simulink model "Lidar_System_July11_PrintV2_Angle_Offset_Bayes_Sunny"  (Simulink 7.3)
settings: Solver=FixedStepDiscrete  StartTime=0.0  StopTime=inf  FixedStep=0.1  MaxStep=0.2  RelTol=1e-3
undefined symbols (not defined in the file): strel
libraries: dspmtrx3 x9, dspstat3 x4, simulink x3, vipstatistics x2, vipgeotforms x1, vipmorphops x1
(part 2 of 5)

== matlab function Enabled Subsystem1/Data Save Interpolation and Bayes/Bayes Filter FSM/RG Speedgate Bayes Filter ==
  data: Task input double; HMean input double; ColorProb output double; SMean input double; VMean input double; ColorNum output double
function [ColorProb, ColorNum] = BayesFilter(Task, HMean, SMean, VMean)
%Written by Anderson Lebbad on June 20, 2014
%Last Edited: by Michael Benson on 7/8/2014 for specific RG task

%Treats the histogram information as a probability distribution of the
%color of an object. Uses the Discrete Bayes Filter with the historgram
%data as measurements, starting without an input.

%initialize a variable to track previous beliefs and one to track number of
%frames iterated upon. Reset every 10 samples

persistent frames
persistent ColorProbabilities

if Task ~= 1
    ColorProb = 0;
    ColorNum = int32(0);
else
    
    if isempty(frames)
        frames = 0;
    end

    if isempty(ColorProbabilities) || frames >= 10
        ColorProbabilities = 1/2*ones(2,1);
        frames = 0;
    end

    %Histogram based probability from reference
    %Filler data from RG A2's
    Red = [0.418812802276720,0,0;0.0194722195087532,0.00139298796126768,5.07737098676741e-05;0.0138492497347506,0.00140176534989290,9.45642160859260e-06;0.0143797281837155,0.00180194953991997,1.58576916205630e-05;0.0159906356383445,0.00122250995735606,2.63324970946963e-05;0.0183249467601919,0.0568841449810760,1.03293220647704e-05;0.0218752453044534,0.00169329388232664,8.72900456177778e-07;0.0234288057788941,0.00992875149521546,9.60190501795556e-06;0.0286071400589464,0.000719431497773991,1.22206063864889e-05;0.0312588481153716,0.00160954411981461,1.97857436733630e-05;0.0305670365822222,0.00550438238362406,8.72900456177778e-06;0.0285293249011251,0.000731557411145066,3.85531034811852e-05;0.0246239069721655,0.00320793785671861,3.15698998317630e-05;0.0190959095363781,0.000679711664623136,4.23356721246223e-05;0.0171575261105718,0.00213992358772399,4.67001744055112e-05;0.0140557162320463,0.000885216251249498,3.52069850658371e-05;0.0120186805075952,0.00203428679112246,2.63324970946963e-05;0.0115340051688313,0.00271600247292672,2.63324970946963e-05;0.0103312647530754,0.00180135945137060,3.97169707560889e-05;0.00954193874440829,0.00147605615682423,3.82621366624593e-05;0.00796761104924986,0.00143910311882922,7.97249083309038e-05;0.00855603843846525,0.00169327353832533,5.95027144294519e-05;0.00739174923569342,0.00121509145857236,6.66491374325861e-05;0.00649026714238162,0.00194416565356162,6.80862355818667e-05;0.00649885840103597,0.00157160944434582,7.20231556068412e-05;0.00596040643778088,0.00194430529700334,5.70294964702815e-05;0.00540944146736658,0.00141314535097839,5.80567483079968e-05;0.00524502462779314,0.00125086331058991,5.86298139732741e-05;0.00558708173689933,0.00146083995084940,5.23740273706667e-05;0.00435272303443563,0.00144723614227691,5.44373990182717e-05;0.00549487305614555,0.00168817541534780,4.43990437722273e-05;0.00368026680360152,0.00159306007523833,6.41936554177648e-05;0.00409020974372935,0.00205652797615577,7.20586274955393e-05;0.00410089139377623,0.00167926242249156,6.27565572684842e-05;0.00326891479557737,0.00159098816892650,6.18091171803395e-05;0.00445211299670090,0.00138590680020840,5.13733794494750e-05;0.00283425405617157,0.00136777016626660,6.32107434409221e-05;0.00309300377822649,0.00140770162395038,6.94243654895015e-05;0.00307199818048493,0.00150035608420383,8.31823221224837e-05;0.00277542868469595,0.00157300356934507,6.40973915794120e-05;0.00278387992211586,0.00154389709907400,0.000110758105837365;0.00229964900594954,0.00164260827201308,7.30152979075107e-05;4.44655768338377e-05,0.00139091758695888,7.48245951759911e-05;0.00889813611845503,0.00158720488030872,8.12400052745627e-05;0.00198142826897388,0.00158792071151883,4.90456448996676e-05;0.00190651941939485,0.00180907399006750,6.19848003607968e-05;0.00225582125348853,0.00165889477609460,7.16381002566071e-05;0.00141288087150997,0.00185423950475477,6.68016758621084e-05;0.00121854137959673,0.00184987366495476,7.80571062129265e-05;0.00869650773841455,0.00198002357227974,7.90613499918661e-05;0.00283670519003113,0.00165854406467308,9.69855100676161e-05;0.0581372528555002,0.00215529068209603,8.89347029816430e-05;0.000223363632106310,0.00212468619148582,4.85581621453762e-05;0.000196405395428911,0.00200335313100036,5.16998181568990e-05;6.12350551728666e-05,0.00191817479458698,5.29736969524676e-05;0.000453580353416284,0.00186497225294572,4.70505126229886e-05;8.46548161411358e-05,0.00190663827294957,5.95825261790225e-05;0.000422587211366844,0.00199789889288887,4.79903685945255e-05;9.51697405110890e-05,0.00221563798239625,5.55643738535741e-05;6.97094055950642e-05,0.00226156124634891,4.37469211133207e-05;0.000352672020849422,0.00250472020727048,4.08346852181048e-05;0.000106693307556525,0.00241527118012696,3.37179629390762e-05;7.61772640109071e-05,0.00258882988304447,2.83021726150822e-05;6.65529572666487e-05,0.00196684177186773,4.15487469837195e-05;8.60084106627102e-05,0.00233772119111424,5.40230353450440e-05;4.93082961912820e-05,0.00227698508497096,6.21985231410858e-05;6.99871626200540e-05,0.00236118701349608,7.77381149267738e-05;4.17810794906234e-05,0.00243959790993590,6.65413012187658e-05;9.43059460511410e-05,0.00262381505622098,6.25955132216168e-05;4.39327384493303e-05,0.00241272700598437,7.11457377921782e-05;6.77317370658152e-05,0.00242356907176823,5.06884893083404e-05;8.80904909050683e-05,0.00234279285042164,4.30549459025671e-05;4.10054710162356e-05,0.00202206116654657,5.70360223908153e-05;5.25969928584074e-05,0.00253828795216140,6.09308079112216e-05;5.98094799256230e-05,0.00250010189524607,6.65882087875949e-05;5.27204786738887e-05,0.00246939421035033,7.97439281308196e-05;5.88503183894037e-05,0.00237587522755561,9.40260932097212e-05;7.13108537607895e-05,0.00239990545025178,8.51284604812913e-05;6.99192479465926e-05,0.00253939132480483,7.10672098981744e-05;6.26092432317400e-05,0.00246119719969018,5.85516484309226e-05;7.76478903519452e-05,0.00256105193836888,7.05681848178752e-05;4.72027776745463e-05,0.00287320739593677,5.61533324585485e-05;6.22308504878448e-05,0.00278061158556548,5.36609880535855e-05;7.84365984049347e-05,0.00319713203504958,3.84505093291548e-05;2.54326892786854e-05,0.00185097795461185,4.59198818278418e-05;0.000151473372383540,0.00271584846618697,3.32438054165253e-05;2.80180039138091e-05,0.00274595292638483,3.93912567519695e-05;5.53332462627916e-05,0.00260298523939083,3.34981354982484e-05;3.61831896348111e-05,0.00263263624778821,3.35821788510691e-05;5.77372432354937e-05,0.00271640119762721,3.17842872132601e-05;5.27135797825679e-05,0.00267032135785430,4.02966389351400e-05;5.05695379036930e-05,0.00268493871523649,3.49858737726195e-05;9.54953413418300e-05,0.00264011882154095,2.89231439463432e-05;6.33501539846335e-05,0.00290170646338386,3.95766693095964e-05;5.50300412672821e-05,0.00283048196980252,4.13286938897529e-05;8.29360851845888e-05,0.00246888746902639,4.71112745231836e-05;3.19810588641323e-05,0.00267918261210111,6.12189501224616e-05;5.23961728497560e-05,0.00274481937827211,6.51297788425716e-05;3.86472632951297e-05,0.00262356594581976,6.53501341892712e-05;5.22572754598462e-05,0.00271370327253989,7.01879791346731e-05;4.60110638382893e-05,0.00275933382763916,7.20086054437621e-05;6.99936331887945e-05,0.00223294619925761,6.72752141398318e-05;6.34334042725368e-05,0.00278169157892946,8.54299279338030e-05;4.38411398324308e-05,0.00279272622079914,8.12459885466860e-05;9.43428590703418e-05,0.00269523707432427,6.17352722085717e-05;4.49809708955904e-05,0.00274871566290032,7.91683701666031e-05;0.000101528135318529,0.00261970779585040,7.44322579682364e-05;4.57463863187916e-05,0.00291387702632575,8.30153401757590e-05;0.000101998442490373,0.00300732388907046,7.40743656836110e-05;8.41092087030208e-05,0.00262624994339149,8.07877210278278e-05;0.000141195946627944,0.00274473037832307,8.91614776125309e-05;0.000127079022997702,0.00270019219328425,8.80237753092585e-05;0.000104131277246489,0.00273021498477153,0.000103968333693197;0.000156109716199346,0.00251020137785535,9.53120858671849e-05;0.000119420105949319,0.00269722007726919,8.52350252231697e-05;0.000153257388529412,0.00244661861602097,6.89965399019053e-05;0.000136609073394080,0.00294979261554324,7.26876177839587e-05;0.000155567767174597,0.00261027159125617,7.14209306975316e-05;0.000113628465885678,0.00285682877063998,8.11734545471175e-05;0.000125949367977156,0.00275960592382486,7.48608642568922e-05;0.000189291966171453,0.00290114176043710,7.82491171704545e-05;0.000210477071818512,0.00278464363993004,6.90690232533521e-05;0.000247727879635590,0.00287502885651961,7.24844091798863e-05;0.000221224323355267,0.00286507033400682,8.56833035452100e-05;0.000247606435361267,0.00305545204943198,6.77579963028754e-05;0.000390223396282197,0.00266116362026216,6.35203500357226e-05;0.000463359252947279,0.00291547128955731,7.05580453769359e-05;0.000316948843843813,0.00135623585761069,7.51642949055405e-05;0.000303566796056351,0.00263290137599010,7.01890497048407e-05;0.000100012530563643,0.00270369869106788,8.81672024349243e-05;0.000144023951274503,0.00267933701167384,8.05940886207993e-05;0.000131935473019354,0.00268146392101225,0.000108123357171141;9.93491089135877e-05,0.00268449853401116,0.000112412291673449;4.11202732797045e-05,0.00259712269173432,0.000117932821400504;3.20593145643942e-05,0.00254079690907548,0.000118166954469444;2.02291422820886e-05,0.00233601609979998,0.000134378972572698;2.05342491905928e-05,0.00270755173260891,0.000141445084785627;1.50928830935123e-05,0.00217625541337369,0.000149639455686249;1.30206434737328e-05,0.00259279807425540,0.000176067021727887;9.38715409422949e-06,0.00230652974475116,0.000174625858736038;7.05055157224756e-06,0.00251745490097623,0.000163270705387633;3.89785228170570e-06,0.00241470223741854,0.000158378761154729;2.65417325723139e-06,0.00252839483583534,0.000146063703891434;5.68799305493382e-06,0.00229740754916477,0.000141062639592320;8.81768428352291e-07,0.00244158084725999,0.000139490994673173;2.57076565309001e-06,0.00219131267591570,0.000130534762983653;1.47257003797866e-06,0.00247860264745366,0.000148967327526605;2.69851311810395e-06,0.00238203133567418,0.000141371960412823;1.37142648948826e-06,0.00200835386214405,0.000151771590515841;0,0.00207035940930703,0.000136619032573913;6.49173263627104e-06,0.00222783724179691,0.000152182536243749;0,0.00211111991830051,0.000142728819044803;1.19933916360175e-06,0.00176935628873998,0.000171308722220559;1.45483409362963e-07,0.00223939320858555,0.000184828783178880;3.03381979770244e-06,0.00217074353330532,0.000183863880543413;1.45483409362963e-07,0.00205145924617477,0.000197484841709011;0,0.00184969041659710,0.000189521008029114;1.18160321925273e-06,0.00203302391019745,0.000185315118782472;0,0.00205057741964801,0.000203145053647263;7.36285018989328e-07,0.00191872611987478,0.000201114234986847;0,0.00227938125138302,0.000195226313365008;3.09949145749479e-06,0.00212336341397899,0.000213486125996751;0,0.00205412921341422,0.000207473566094751;2.99834790900439e-07,0.00185151516359060,0.000207406521624767;8.90636400526803e-07,0.00186248859732819,0.000183341482655647;1.68899722473772e-06,0.00193500038779790,0.000211978261985679;0,0.00199879299929424,0.000196068363552520;0,0.00213005077179156,0.000213310677211431;1.45483409362963e-07,0.00226448101068235,0.000254057130439161;0,0.00157666277757647,0.000266568758413429;0,0.00240265450950301,0.000285630735682664;9.53352895487022e-06,0.00212217380237139,0.000316744144969953;0,0.00217033136797276,0.000347296809278156;0,0.00195155596397510,0.000350819310353655;0,0.00197136585358172,0.000374224667783579;0,0.00197401567470083,0.000333386251171196;0,0.00225727278194117,0.000376045619823585;4.63054144612427e-07,0.00225500699055331,0.000413333437163438;4.54186172437914e-07,0.00206219785523074,0.000407191651543640;2.99834790900439e-07,0.00214402826730192,0.000456285295707928;0,0.00210716655790327,0.000463388104092460;9.08372344875829e-07,0.00224111576073664,0.000492907406114772;0,0.00170207435823317,0.000490017162461332;7.71756907687378e-07,0.00207988071440082,0.000479532398573352;0,0.00201065397987837,0.000516543874663399;2.98947993682987e-06,0.00199450170188781,0.000464866534941865;0,0.00177671736127319,0.000469246302623159;1.45483409362963e-07,0.00189175987991769,0.000527230176751719;1.54351381537476e-07,0.00187401189637039,0.000600250030866361;9.26108289224854e-07,0.00200277400075776,0.000514808246628158;0,0.00197953547678507,0.000562698936262369;0,0.00155455061017225,0.000572964589360564;4.22518244040745e-06,0.00198779350468226,0.000523625276904511;0,0.00200076476505620,0.000616447190540555;1.54351381537476e-07,0.00176354543818283,0.000642568677493060;0,0.00201458246429843,0.000632021564242528;9.26108289224854e-07,0.00198485552332751,0.000689386452587112;0,0.00188631273418289,0.000684597701362130;0,0.00194984914991706,0.00104741783900229;2.41641427155253e-06,0.00186793794617886,0.00100164960594678;0,0.00189473075595684,0.000959830770760674;3.08702763074951e-07,0.00190594993204555,0.00112452932795823;0,0.00194085676172101,0.00101608491830048;1.31821865644118e-06,0.00170847754263923,0.00108169844026045;0,0.00198170260629892,0.00105383542393514;3.08702763074951e-07,0.00210488869443961,0.00102225981496908;4.63054144612427e-07,0.00196488951978371,0.00142330496824817;1.54351381537476e-07,0.00196396824180039,0.00140267367413510;0,0.00190308572363885,0.00120878275630225;0,0.00187071228421696,0.00205322784788965;0,0.00198115641717238,0.00173893426378925;0,0.00208977844254468,0.00188806599530812;0,0.00179340738821397,0.00167046248806787;1.24298418641064e-05,0.00218935197268131,0.00275908125480616;0,0.00192774256781834,0.00157355834898318;0,0.00204901563154405,0.00350939920376686;0,0.00202326008635860,0.00632085665053410;0,0.00213558501768675,0.00669789463168136;1.08045967076233e-06,0.00207714353839267,0.00627563514000161;0,0.00225995513740419,0.00250544981401045;1.45483409362963e-07,0.00223563601660356,0.00628662925532504;0.000107410825605734,0.00228770076342562,0.00694054742809225;2.13431542500112e-06,0.00225603417304346,0.00563315640424600;2.90966818725926e-07,0.00220257190544410,0.00749520898429996;2.67190920158041e-06,0.00222918142788297,0.0101271846978441;2.99834790900439e-07,0.00234595332802456,0.00694290376571382;1.49030598232768e-06,0.00229601957392332,0.0129468824474908;8.90636400526803e-07,0.00258945498766694,0.0159801589818961;4.27093165619752e-05,0.00230717065782069,0.0150667035339748;1.31821865644118e-06,0.00237610367689422,0.0144312222281109;3.11722740184381e-06,0.00240501038018950,0.0387860160710828;6.85186032983753e-06,0.00230587982511823,0.0142080286927282;5.00851172356233e-06,0.00240837658981136,0.253900841876681;4.50998569025186e-06,0.00258880916558226,0.0183449808209977;4.99964375138782e-06,0.00265683863733496,0.0144575158948879;3.75555647575547e-05,0.00342846223898661,0.0170167582050570;1.74294856154943e-05,0.00331827817329332,0.0171418698632039;1.37299321687324e-05,0.00339160394932691,0.0174772463377933;1.16501084323452e-05,0.00383120615703546,0.0178604644454266;2.10577028773938e-05,0.00404692001829078,0.0196329380603643;2.43128295719929e-05,0.00436779279654884,0.0212313110641294;4.08217347279958e-05,0.00609041339337509,0.0228963122790907;3.85503035932928e-05,0.00632406275849346,0.0227626430174866;2.26835183505936e-05,0.00663320374789515,0.0254917960021599;3.32935187110122e-05,0.0156813466261263,0.0244074642420541;4.90044365398483e-05,0.0242377204839236,0.0238488375177945;3.74385382082969e-05,0.0254873378699169,0.0202960165575666;3.70503572106603e-05,0.287237951700180,0.0201973404850723;5.25056022033951e-05,0.00590919265813658,0.0192098345312769;9.09691580564597e-05,0.0135465726949558,0.0195085996911853;0.000121508740524264,0.00247847860111233,0.0161886324548659;0.000301689558076566,0.00212561673317700,0.0147470760761275;0.000480987078225832,0.00136429432132458,0.0153705482830582;0.00116738829366397,0.00105211487702614,0.0727297039365956;0.0112209100765555,0.00644597379873206,0.0532084254345464;0,0,0];
    Green = [5.64759498395346e-05,0,0;8.59416627992918e-06,2.45547607997977e-05,0;1.90299396198432e-05,0.000189685527178437,0;7.55058894593778e-05,0.00117801464937029,6.13869019994942e-07;0.000150397909898761,0.000844683771513040,0;9.14664839792463e-05,0.00123633220626981,3.68321411996965e-06;0.000142417612638826,0.00105892405949127,4.29708313996459e-06;0.000142417612638826,0.000675255921994436,2.51686298197926e-05;0.000230200882498103,0.000716999015354092,2.94657129597572e-05;5.58620808195397e-05,0.000726207050654016,7.61197584793728e-05;0.000174952670698558,0.000755672763613773,3.37627960997218e-05;0.000307548379017466,0.000762425322833718,4.54263074796257e-05;0.000289420246980742,0.000736028954973935,3.58923417228313e-05;0.000283281556780793,0.000649473423154648,3.83478178028111e-05;0.000301947574050020,0.000649473423154648,4.87835911427251e-05;0.000237779265513676,0.000776544310293601,3.40507346628465e-05;0.000173361010307953,0.000828109307973176,7.42401595256423e-05;0.000331261319434795,0.000915892577832453,5.21788666995701e-05;0.000165804622599285,0.000850822461712989,0.000112799932104087;0.000142515591733223,0.000728662526733996,0.000107964963731619;0.000126077099181502,0.000774088834213622,0.000156172677748094;0.000280310190775215,0.00100981453789168,0.000176104424951057;0.000179141776877351,0.00102884447751152,0.000198567632021491;0.000183416864710410,0.000995081681411801,0.000159893883761809;0.000187561980275393,0.000963160492372064,0.000188093866787831;0.000176126420257962,0.000984645908071887,0.000233808112830582;0.000169699791494888,0.000979121086891932,0.000234134043287452;0.000165152761685545,0.000940447338632251,0.000341735084668454;0.000275899131954013,0.00103158789215463,0.000340545338522210;0.000205804087993353,0.000976627618918207,0.000348085729644037;0.000196997966937790,0.000945858184130968,0.000355028248332710;0.000167972160116140,0.000945532253674098,0.000319885746618016;0.000253761855340450,0.00109054131338105,0.000496392085813434;0.000193102798042187,0.00119077592652211,0.000510571060473969;0.000251958240174211,0.000954822271481579,0.000559756565861055;0.000292821521257652,0.00100104240958315,0.000399460767854884;0.000216603783683883,0.000802262822786028,0.000345462289402235;0.000247433205671772,0.00112734746012713,0.000326954238428055;0.000271374097451575,0.00105585071524459,0.000470067702594433;0.000214132311017063,0.000976313685901467,0.000380170883698887;0.000255799420589228,0.00102051225534110,0.000468302079321939;0.000195814219511611,0.00120690048605709,0.000382262437428251;5.46343427795498e-05,0.00122639232712195,0.000474576740510031;0.000634540609339266,0.00120941594933772,0.000488929678052453;0.000230402839406961,0.00127995089943649,0.000496432077280535;0.000306788541142554,0.00139554823466427,0.000576544983749907;0.000232276439640627,0.00107708018555497,0.000476190396207542;0.000381278647337575,0.00125351054096290,0.000658461505385519;0.000403187972588665,0.00128177051118957,0.000565849265873839;0.000451873584636993,0.00120901803424007,0.000655072228548739;0.000473472976018053,0.00147160200722292,0.000658733447361803;0.000478671866741137,0.00150686448333892,0.000719778422317587;0.000394169896757469,0.00146907654607552,0.000708184896005109;0.000446984627783939,0.00155343254720427,0.000867698860829463;0.000383484176748176,0.00165554675929906,0.000687889226451530;0.000318300084947475,0.00148379340596856,0.000647765787509451;0.000330577465347374,0.00148435928522803,0.000645038369453187;0.000727000881275964,0.00169511231727509,0.000608924075087947;0.000416845058603536,0.00166131752800169,0.000503936476081971;0.000389872813617504,0.00179897215690882,0.000514638192678105;0.000464476895493762,0.00182383685157865,0.000661174926428298;0.000589940125655269,0.00182472266257493,0.000630039569717089;0.000625148613290679,0.00182507258791206,0.00100136834004002;0.000750883785428471,0.00159226826090571,0.000557341081248176;0.00109448847118388,0.00189448977650537,0.000580316179097498;0.000913545078713645,0.00207851651108906,0.000418236761658638;0.00103039814600838,0.00216843532529151,0.000525267924633457;0.00123675611582108,0.00226885989790130,0.000374706049719583;0.00168685807846551,0.00262634762146070,0.000329915606566858;0.00210315525396977,0.00263831906713728,0.000310559736490145;0.00238629284146900,0.00270115366024582,0.000276606980921695;0.00273374270678614,0.00255027185359514,0.000275705173338575;0.00279548953198954,0.00267357354495986,0.000320599594305762;0.00372449131273758,0.00295677911795316,0.000381584582060895;0.00487414401364010,0.00298961411201615,0.000429814291384276;0.00514913134014422,0.00286661635580140,0.000472975082252650;0.00569852411730614,0.00282401944461914,0.000615186738835908;0.00815310038927614,0.00330093168680785,0.000720202331868854;0.0107508621100533,0.00271035769639904,0.000653366592476897;0.0115851920907340,0.00328122189224730,0.000633918742025852;0.0129208710995752,0.00336854725980827,0.000759473952561690;0.0153363777077613,0.00311447946974450,0.000764488882536111;0.0193231670544919,0.00336194266901660,0.000708648797023477;0.0214687792495091,0.00330959383858185,0.000838291135497001;0.0255558092081009,0.00254408917278138,0.000688787034887940;0.0774038724905344,0.00347457663653222,0.000884309316689717;0.0413451982577381,0.00313356339784493,0.000861360213294010;0.0338858518435638,0.00356296577711807,0.000977741381276960;0.0301487272263692,0.00324231019475837,0.000817907484715801;0.0306436356287532,0.00325953451963861,0.00108866371400067;0.0332230312682644,0.00367098872847698,0.00111743557500623;0.0374729024817433,0.00364719180597874,0.00113174852108155;0.0397526880484565,0.00340957450590682,0.00121187742413777;0.0378740048993227,0.00349219087821670,0.00114813702429940;0.0324405302289461,0.00340957050676011,0.00135120969508978;0.0290666781010269,0.00342488923823302,0.00136713029814255;0.0296407496125367,0.00402534911930911,0.00145728906114760;0.0356849959637812,0.00483235493009328,0.00157320432853883;0.0395630245165850,0.00437495852384968,0.00216359435819898;0.0407753598430210,0.00424826955522154,0.00160306195787617;0.0380115275563884,0.00498365264800180,0.00154762978532796;0.0368282500299476,0.00354253613614970,0.00173022282581610;0.0298285795356416,0.00453824568359498,0.00184178502201342;0.0210234802620634,0.00409398047557389,0.00244841958560986;0.0164048057394090,0.00364579410420357,0.00298893225750208;0.0110889379754820,0.00403142982188177,0.00338672938032558;0.00908992650056243,0.00426539990015410,0.00347458863397235;0.00814236268035962,0.00379832955801887,0.00359348926438264;0.00720789806520562,0.00399952462942887,0.00441631969869853;0.00639686311411107,0.00335357445452579,0.00372866442232954;0.00608482769248491,0.00376550256224930,0.00491582312065239;0.00572428861998573,0.00361931575383624,0.00333207504181248;0.00615469278550974,0.00392753598950099,0.00435011382491341;0.00583404720101681,0.00396643968869650,0.00353824505172980;0.00481320501607213,0.00425503011273491,0.00490912654948639;0.00461989626197437,0.00435664443149094,0.00484768765857967;0.00432509116394853,0.00436277512339747,0.00482097135898308;0.00428296615207806,0.00417634890078774,0.00561831723088908;0.00444561344834975,0.00412345618640042,0.00479221749413771;0.00485890926424811,0.00399275807319544,0.00541906774435352;0.00455306652130248,0.00426289643431360,0.00456264647724644;0.00445239200202331,0.00371740082562064,0.00514094308725536;0.00292324427321591,0.00381317639017998,0.00458484774020737;0.00228359275438118,0.00371428549033350,0.00516145271115793;0.00206628312130297,0.00351831730367355,0.00523129580887585;0.000976665610811952,0.00422639422271749,0.00480587058100587;0.000291587784497597,0.00461505529488184,0.00559332656309789;7.91891035793475e-05,0.00283711465052125,0.00483196501328904;8.53277937792969e-05,0.00437326288564462,0.00601825789634917;1.22773803998988e-06,0.00408650607037278,0.00495514673025246;5.52482117995448e-06,0.00400633717584946,0.00554387111530787;2.51686298197926e-05,0.00408818171284429,0.00567739662523687;2.27131537398128e-05,0.00398538764580879,0.00608597144844399;6.75255921994436e-06,0.00380842940303513,0.00558363463104604;9.20803529992413e-06,0.00384641129891397,0.00604918729700481;9.20803529992413e-06,0.00372969820175409,0.00621786330694192;9.20803529992413e-06,0.00400794083368020,0.00606026093424498;6.75255921994436e-06,0.00380664578360244,0.00669104834439685;4.91095215995953e-06,0.00358835036086020,0.00605819537496923;3.06934509997471e-06,0.00360229738501155,0.00596688685728503;6.13869019994942e-07,0.00382027287601699,0.00535548930995691;1.22773803998988e-06,0.00353426790032664,0.00576435607087387;0,0.00335357845367250,0.00644283730468997;0,0.00337721740987569,0.00604661584567024;6.13869019994942e-07,0.00348590621916183,0.00699461157371774;0,0.00342531714693099,0.00635565390683721;0,0.00372344753544626,0.00619957920818351;0,0.00347543045435482,0.00658468703849597;0,0.00366662365984295,0.00592171649519485;0,0.00356604711965817,0.00645419688091991;1.22773803998988e-06,0.00406898380906263,0.00567350145634126;0,0.00448059198504933,0.00693635800316558;0,0.00382477591521252,0.00621570576729184;0,0.00485564995967940,0.00668098449170098;0,0.00517649750108119,0.00584956788939857;0,0.00467551439484460,0.00502189248884344;0,0.00470294254255558,0.00603507630783835;6.13869019994942e-07,0.00552914425754806,0.00536562514729357;0,0.00472664748467949,0.00753366455706079;0,0.00517075072725883,0.00610449549600501;0,0.00517506380698563,0.00765498067208396;0,0.00434342525204082,0.00595371766716879;0,0.00474935463969924,0.00645238526746025;0,0.00471952700396222,0.00584119767533441;0,0.00432027819088297,0.00574709575367323;0,0.00484209285233228,0.00581612102588895;0,0.00462894233183254,0.00493404123349009;0,0.00456246051692442,0.00575447817850001;0,0.00473505769021076,0.00554162559443017;0,0.00386035432391861,0.00732101193032645;0,0.00599809619821038,0.00634392640910994;0,0.00479977788099309,0.00704802417717736;0,0.00466920774048283,0.00625805473137808;0,0.00440997905158972,0.00624668115813465;0,0.00465340111311130,0.00624744699472963;0,0.00439547214689896,0.00589866341398469;0,0.00439056919303242,0.00600098558170840;0,0.00443649139470410,0.00569505485753516;0,0.00431867253347888,0.00691925765183334;0,0.00421240320795233,0.00662945348676844;0,0.00467333485988762,0.00705019171469422;0,0.00447672281060735,0.00597042010340338;0,0.00395828742812804,0.00623599143897865;0,0.00482459858504911,0.00539866009869206;0,0.00454055319124669,0.00583414118096450;0,0.00432886035972277,0.00486946501198932;0,0.00410780752532394,0.00582520308806751;0,0.00422122332602137,0.00548064260624839;0,0.00439713979107706,0.00544155894545093;0,0.00428031071866258,0.00533965668813177;0,0.00470300053018288,0.00525706830984886;0,0.00393274687766421,0.00520099427425369;0,0.00555682835064848,0.00487591563563266;0,0.00457001690463309,0.00531875714742497;0,0.00420474884114926,0.00495514273110575;0,0.00465595856743238,0.00519652322823184;0,0.00463093190732080,0.00500288454453050;0,0.00492873236623248,0.00567429128781650;0,0.00419772034080632,0.00489002262565241;0,0.00421868386786048,0.00526393884389676;0,0.00511469268825049,0.00488106053787516;0,0.00526538453543245,0.00467656817000270;0,0.00490855467150685,0.00456539389103626;0,0.00345000987829229,0.00406302308089128;0,0.00462860640350890,0.00453736787089212;0,0.00456198261889257,0.00404162364684572;0,0.00493546293014552,0.00444073448936347;0,0.00467908963200340,0.00422475257299301;0,0.00431227789788948,0.00444271006783825;0,0.00409613001693055,0.00467503049809268;0,0.00461236786829268,0.00474394579377387;0,0.00445775885690822,0.00499614998147075;0,0.00446023832786846,0.00474439969692547;0,0.00442528378604914,0.00438825968580736;0,0.00448351736086775,0.00423129117786396;0,0.00422702608789768,0.00380091500636692;0,0.00387561106861751,0.00360495081885368;0,0.00415454955207117,0.00351548590780282;0,0.00432765461698968,0.00405649247431374;0,0.00442837912560273,0.00426218858534592;0,0.00455286256482027,0.00456368025667100;0,0.00571846186322917,0.00474052852291012;0,0.00489332192168821,0.00501781735834589;0,0.00554325124756781,0.00511884980125561;0,0.00539161360218893,0.00499287468031521;0,0.00647129923182551,0.00466519459675928;0,0.00636939897407970,0.00441318636725119;0,0.00595304181137479,0.00406295109625050;0,0.00726374015029161,0.00375835808665177;0,0.00718969594895476,0.00381996294214696;0,0.00701155595832828,0.00382337621386400;0,0.00928017990657369,0.00394267875851865;0,0.0100841063743911,0.00444330794027140;0,0.0117657975553072,0.00452831980146060;0,0.0148302077082417,0.00453800173564567;0,0.0193894089205974,0.00453077327796723;0,0.0178914325408216,0.00495280522985372;0,0.0176311900682375,0.00464262341272767;0,0.0178718387215157,0.00506823460091967;0,0.0170407240547899,0.00615487874583176;0,0.0155849946608592,0.00678355260694736;0,0.0125271870991430,0.00828430839368666;0,0.0100083805318627,0.00895988224784454;0,0.00969168610431929,0.0101424999150781;0,0.00543921344590547,0.0115618850637077;0,0.00547018083845486,0.0133732605741378;0,0.00277857314140596,0.0144005813767528;0,0.00380991708561128,0.0166686794372058;0,0.00173858704116020,0.0182121861022757;0,0.00213851570918016,0.0186627399684984;0,0.00181987169761562,0.0195606703788826;0,0.00113063075957609,0.0184694192169605;0,0.00161016844157996,0.0154263585087377;0,0.000453611213882516,0.0122882820738305;0,0.0290299159448947,0.0333400223061206;0,0,0];
    

    RedH = Red(:,1);
    RedS = Red(:,2);
    RedV = Red(:,3);
    GreenH = Green(:,1);
    GreenS = Green(:,2);
    GreenV = Green(:,3);

    %Combine probs into channel matrices
    ProbH = [RedH, GreenH];
    ProbS = [RedS, GreenS];
    ProbV = [RedV, GreenV];

    %No input, 2 measurements, 2 states
    for i=1:2
        ColorProbabilities(i) = (ProbH(HMean+1,i)*ProbS(SMean+1,i)*ProbV(VMean+1,i))*ColorProbabilities(i);
    end

    %Sum for normalization
    TotalProb = sum(ColorProbabilities);

    %Update frame count
    frames = frames + 1;

    %Check to make sure ColorProbabilities has values, if so normalize
    if (TotalProb == 0)
        ColorProbabilities = 1/2*ones(2,1);
        frames = 0;
    else
        %Normalize
        ColorProbabilities = ColorProbabilities/TotalProb;
    end



    %Output - First element is red prob, then green prob
    [OrderedProbs, Order] = sort(ColorProbabilities,'descend');
    ColorProb = OrderedProbs(1);
    %ColorProb = 0.6;
    ColorNum = int32(Order(1));
end

== matlab function Enabled Subsystem1/Data Save Interpolation and Bayes/Template Matching Subsystem/Detection/Detection ==
  data: cruciform input double; bbox_out output double; circle input double; triangle input double; whitePixCount input double; threshold input double; V_mask input double; bbox_in input double; label input double; rtnRatioDiff output double
function [bbox_out,rtnRatioDiff]= detection(cruciform,circle,triangle,...
    whitePixCount,threshold,V_mask,bbox_in,label)

% Written by Edward Zhu on 5/14/14
% Last Edited by Anderson Lebbad on 7/10/14 - adapted for r2009a

% Inputs
% tempID:       Number corresponding to one of the templates (cruciform: 1,
%               circle: 2, triangle: 3)
% cruciform:    19*19 template of cruciform
% circle:       19*19 template of circle
% triangle:     19*19 template of triangle
% whitePixCount:Number of white pixels in each of the templates
% V_mask:       V channel binary mask
% bbox_in:      Bounding boxes as found by blob analysis
% label:        Label matrix as found by blob analysis

% Outputs
% bbox_out:     Bounding box of matched symbol
% symFound:     Status of matching (found: 1, not found: 0)

% Define frame and template size
templates = zeros(19,19,3);
templates(:,:,1) = cruciform;
templates(:,:,2) = circle;
templates(:,:,3) = triangle;

imgRows = size(label,1);
imgCols = size(label,2);
tempRows = size(templates,1);
tempCols = size(templates,2);
numBBox = size(bbox_in,2);

% Initialize scaled image and output bbox matrices
V_scaled = zeros(tempRows,tempCols);
bbox_out = uint32(zeros(4,numBBox));
rtnRatioDiff = ones(numBBox,1);

bestRatioDiff = single(1);

for i = 1:numBBox
    shapeDiff = abs(1-bbox_in(4,i)/bbox_in(3,i));
    if bbox_in(4,i) >= tempCols && bbox_in(3,i) >= tempRows && shapeDiff < 0.5
        % Set up arrays for the start and end rows and columns for bbox
        % matching
        
        similarity = zeros(1,3);
        ratioDiff = zeros(1,3);
        
        rowStep = floor(bbox_in(3,i) / tempRows);
        colStep = floor(bbox_in(4,i) / tempCols);
        
        startRowList = zeros(1,3);
        startRowList(2) = bbox_in(1,i)+1;
        startRowList(1) = max(1, startRowList(2) - rowStep);
        startRowList(3) = min(imgRows, startRowList(2) + rowStep);
        
        endRowList = zeros(1,3);
        endRowList(2) = bbox_in(1,i)+1 + bbox_in(3,i);
        endRowList(1) = max(1, endRowList(2) - rowStep);
        endRowList(3) = min(imgRows, endRowList(2) + rowStep);
        
        startColList = zeros(1,3);
        startColList(2) = bbox_in(2,i)+1;
        startColList(1) = max(1, startColList(2) - colStep);
        startColList(3) = min(imgCols, startColList(2) + colStep);
        
        endColList = zeros(1,3);
        endColList(2) = bbox_in(2,i)+1 + bbox_in(i,3);
        endColList(1) = max(1, endColList(2) - colStep);
        endColList(3) = min(imgCols, endColList(2) + colStep);
        
        % Scale down image in bbox to size of template (18*18 px)
        for startRow = startRowList
            for endRow = endRowList
                rowScaleStep = floor((endRow - startRow) / tempRows);
                
                for startCol = startColList
                    for endCol = endColList
                        colScaleStep = floor((endCol - startCol) / tempCols);
                        
                        captureRow = startRow;
                        for row = 1:tempRows
                            captureCol = startCol;
                            for col = 1:tempCols
                                V_scaled(row,col) = V_mask(captureRow,captureCol);
                                for tempID = 1:3
                                    similarity(tempID) = similarity(tempID) + templates(row,col,tempID) * (V_mask(captureRow,captureCol)*(-1) + 1);
                                end
                                captureCol = captureCol + colScaleStep;                        
                            end
                            captureRow = captureRow + rowScaleStep;
                        end                  
                        
                        for tempID = 1:3   
                            ratioDiff(tempID) = abs(1 - single(similarity(tempID)) / single(whitePixCount(tempID))); 
                        end
                        
                        if min(ratioDiff) < bestRatioDiff
                            bestRatioDiff = single(min(ratioDiff));
                        end
                    end
                end
            end
        end
        
        % Output valid bounding boxes
        if bestRatioDiff < threshold
            bbox_out(:,i) = bbox_in(:,i);
            rtnRatioDiff(i) = bestRatioDiff;
        end
    end
end

== matlab function Enabled Subsystem1/Data Save Interpolation and Bayes/Raster to UV ==
  data: uv_d output double; dist_im input double
function uv_d   = AngleMatch( dist_im )
%Written by Anderson Lebbad on July 8, 2014
%Last Edited: by Anderson Lebbad on July 11, 2014

%This function infers depth locations into a image plane based upon the
%angles as they relate to the field of view of the camera. This works
%decently, but loses accuracy at closer ranges as the spacial translation
%between the video camera and lidar becomes more noticeable

%% Initialize

uv_d = zeros(120,160);

%% Parameters

%Camera field of view to determines indices to match
FoVx = 62;
FoVy = 46;

%Scan angles for lidar gimbal
upAngle = 30;
downAngle = -45;
angleRange = upAngle-downAngle;

%Offset angles to account for difference of perspective
HighOffset = 8;
LowOffset = 4;
OffsetStep = (HighOffset-LowOffset)/(120-1);
n1Offset = HighOffset:-OffsetStep:LowOffset;

%% Operation


% Depth frame, same aspect ratio as image frame, quarter width and height
for i = 1:160
    for j = 1:120
        % Effective coordinate in pixel frame
        u = (i-1)/(160-1)*(640-1)+1;
        v = (j-1)/(120-1)*(480-1)+1;
        
        % Scan angle for pixel location being analyzed in degrees
        scanAngleHoriz = -FoVx/2 + (u-1)*FoVx/(640-1);
        scanAngleVert = FoVy/2 - (v-1)*FoVy/(480-1) - n1Offset(j);
        
        % Estimate closest scan value for pixel being evaluated
        xCenter = round((67.5+scanAngleHoriz)*(540-1)/135+1);
        yCenter = round((upAngle-scanAngleVert)*(65-1)/(angleRange)+1);
        
        % Assign
        uv_d(j,i) = dist_im(yCenter,xCenter);
    end
end

end

== matlab function Enabled Subsystem1/Data Save Interpolation and Bayes/Template Matching Subsystem/Recognition/Recognition ==
  data: targetTemp input double; cruciform input double; bbox_out output double; circle input double; triangle input double; whitePixCount input double; threshold input double; V_mask input double; bbox_in input double; returnRatioDiff output double
function [bbox_out,returnRatioDiff] = recognition(targetTemp,cruciform,circle,triangle,...
    whitePixCount,threshold,V_mask,bbox_in)

% Written by Edward Zhu on 5/14/14

% Inputs
% tempID:       Number corresponding to one of the templates (cruciform: 1,
%               circle: 2, triangle: 3)
% cruciform:    19*19 template of cruciform
% circle:       19*19 template of circle
% triangle:     19*19 template of triangle
% whitePixCount:Number of white pixels in each of the templates
% V_mask:       V channel binary mask
% bbox_in:      Bounding boxes as found by blob analysis
% label:        Label matrix as found by blob analysis

% Outputs
% bbox_out:     Bounding box of matched symbol
% symFound:     Status of matching (found: 1, not found: 0)

% Define frame and template size
templates = zeros(19,19,3);
templates(:,:,1) = cruciform;
templates(:,:,2) = circle;
templates(:,:,3) = triangle;
templates = 2*(templates-0.5);

tempRows = size(templates,1);
tempCols = size(templates,2);
numBBox = size(bbox_in,2);

% Initialize scaled image and output bbox matrices
V_scaled = zeros(tempRows,tempCols);
bbox_out = uint32(zeros(4,numBBox));

returnRatioDiff = ones(numBBox,1);

for i = 1:numBBox
    if min(bbox_in(:,i)) >= 0
        similarity = 0;
        rowScaleStep = floor(bbox_in(3,i) / tempRows);
        colScaleStep = floor(bbox_in(4,i) / tempCols);
        
        captureRow = bbox_in(1,i)+1;
        for row = 1:tempRows
            captureCol = bbox_in(2,i)+1;
            for col = 1:tempCols
                V_scaled(row,col) = V_mask(captureRow,captureCol);
                similarity = similarity + templates(row,col,targetTemp) * (V_mask(captureRow,captureCol)*(-1) + 1);
                captureCol = captureCol + colScaleStep;
            end
            captureRow = captureRow + rowScaleStep;
        end
        
        ratioDiff = abs(1 - single(similarity) / single(whitePixCount(targetTemp)));
        
        % Output valid bounding box
        if ratioDiff < threshold
            bbox_out(:,i) = bbox_in(:,i);
            returnRatioDiff(i) = ratioDiff;
        end
    end
end

== matlab function Enabled Subsystem1/Data Save Interpolation and Bayes/Template Matching Subsystem/Bay Position ==
  data: xRec input double; bayNumber output double; xDet input double
function bayNumber = bayPosition(xRec,xDet)

symxpos = xRec(1);

if size(xDet,2) == 3
    diff1 = xDet(1) - symxpos;
    diff2 = xDet(2) - symxpos;
    diff3 = xDet(3) - symxpos;
    
    if diff1 == 0
        bayNumber = uint8(1);
    elseif diff2 == 0
        bayNumber = uint8(2);
    elseif diff3 == 0
        bayNumber = uint8(3);
    else
        bayNumber = uint8(0);
    end
    
else
    bayNumber = uint8(0);
end

== matlab function Enabled Subsystem1/Data Save Interpolation and Bayes/Embedded MATLAB Function1 ==
  data: bbox input double; HMean output double; BW input double; uv_d input double; H input double; S input double; V input double; SMean output double; VMean output double; DMean output double; Angle output double
function [HMean, SMean, VMean, DMean, Angle] = bbox_hist(bbox, BW, uv_d, H, S, V)
%This function creates a histogram of the color region of a detected object
%identified in a binary image within a bounding box

%Initialize variables
pixels = 0;
DRunAve = 0;
HRunAve = 0;
SRunAve = 0;
VRunAve = 0;
FoV = 62;

%Parse bbox data
left = bbox(2) + 1;
right = left + bbox(4) - 1;
bottom = bbox(1) + 1;
top = bottom + bbox(3) - 1;
Angle = int32((double(left) + double(bbox(4))/2-320)/320*FoV/2);

%Check to see if valid bbox is found
if left~=-1
    %Scan the detected region of the binary image and generate histograms
    for j=left:right
        for i=bottom:top
            if BW(i,j) == 1
                pixels = pixels + 1;
                DRunAve = ((pixels-1)/pixels)*DRunAve + (1/pixels)*double(uv_d(i,j));
                HRunAve = ((pixels-1)/pixels)*HRunAve + (1/pixels)*double(H(i,j));
                SRunAve = ((pixels-1)/pixels)*SRunAve + (1/pixels)*double(S(i,j));
                VRunAve = ((pixels-1)/pixels)*VRunAve + (1/pixels)*double(V(i,j));
            end
        end
    end
    %CDist = uv_d(left,right);
end

%Means must be integers to use in Bayes Filter
DMean = int32(DRunAve/10);
%DMean = int32(CDist);
HMean = uint8(HRunAve);
SMean = uint8(SRunAve);
VMean = uint8(VRunAve);

end

== matlab function Enabled Subsystem1/Data Save Interpolation and Bayes/Lidar Image Creator ==
  data: lidarData input double; dist_image output double; UpDown input double
function dist_image = scanImages(lidarData,UpDown)
%Written by Anderson Lebbad on July 5, 2014
%Last Edited:

%Converts the one dimensional array of lidarData and the scan settings into
%frames of distances and angles for each point

% Set output sizes
dist_image = zeros(65,540);

% To run through the middle half of the points horizonatal points, the
% first quarter must be skipped (of 1080)
scanOffset = 270-1;

% Loop through all points in output matrices
for j=1:540
    for i=1:65
        % Select the lidarData that will be used in analysis and format as
        % a frame
        dist_image(i,j) = lidarData(j+scanOffset+1080*(i-1));
    end
end

% Flip if up scan
if UpDown
    dist_image = flipud(dist_image);
end

dist_image = fliplr(dist_image);

end

== matlab function Enabled Subsystem1/Data Save Interpolation and Bayes/Lidar data selector ==
  data: lidarIn input double; lidarOut output double
function lidarOut = data_selector(lidarIn)
% Lidar data is always input as a 1x70200 matrix.
% If Scan Number is less than 65 some of this data may be blank
% Select only the parts of the matrix where data has been collected

FullLength = 1080*65;
DataLength =  1080*65;
lidarOut = zeros(FullLength,1);

% ClosePts = (lidarIn < 3);
% lidarOut = (lidarIn + 30000*ClosePts)/10;

for i = 1:DataLength
    if (lidarIn(i,1) < 3)
        lidarIn(i,1) = 30000;
    end
    lidarOut(i,1) = lidarIn(i,1);
end

%lidarOut = lidarIn(1,1:DataLength);

== matlab function Enabled Subsystem1/Data Save Interpolation and Bayes/Task Parse ==
  data: Task input double; TemplateEn output double; TargetTemplate output double
function [TemplateEn, TargetTemplate] = TaskParse(Task)
%Written by Anderson Lebbad on July 10, 2014
%Last Edited:

%The task signal passes both current task and target template information,
%so this function checks to see if any of the template based task numbers
%are selected, and passes which template the number is associated with as
%well as enables the template matching subsystem.


%Template matching task #s: are 7 (circle), 8 (cruciform) and 9 (triangle)
if Task >= 7
    TemplateEn = 1;
    %Target template #s are 1 (circle), 2 (cruciform) and 3 (triangle)
    TargetTemplate = uint32(Task - 6);
else
    TemplateEn = 0;
    %Really just a filler value, shouldn't matter since subsystem is
    %disabled anyway
    TargetTemplate = uint32(1);
end

== matlab function Enabled Subsystem1/Embedded MATLAB Function ==
  data: potVal input double; yn output double
function yn = check_pot_val(potVal)
%#eml

% Pot value may initially be zero.
% Check for this and output a 1 or zero to 
% control whether the rest of model runs
if (potVal == 0)
    yn = 0;
else
    yn = 1;
end

== matlab function Enabled Subsystem1/Stepper Speed and Postion Calculation ==
  data: UpAngle input double; Speed output double; DownAngle input double; Upos output double; Dpos output double; ScanNum output double
function [Speed,Upos,Dpos,ScanNum] = stepper_calc(UpAngle,DownAngle)
% Last Edited by Anderson Lebbad on July 7, 2014
% edits were made to account for new calibration on gimbal

% This function inputs desired positive and negative scan angles
% and desired number of scans and outputs results positions for
% the stepper and the required speed of the stepper motor to properly
% move so the desired number of scans is obtained over the course of
% the motion of the stepper

% Scan Number requires no change
ScanNum = 65;
% Number of steps for 180 degree flip
stepRes = 3950;
% Parameter to account for slack in the gears with respect to steps
stepGive = 57;

% Transformation of angle to stepper position obtained from stepper calibration
% Output must be an integer
% 57 is added or subtracted due to wobble of gimbal system
Upos = round(UpAngle*stepRes/180)-stepGive;
Dpos = round(DownAngle*stepRes/180)+stepGive;

% Transformation of speed based 
% Output must be an interger
Speed = round(abs(UpAngle-DownAngle) * (1214/90));
